simulink model "sf_cruise_control_test"  (R2017b)
settings: Solver=ode45  StartTime=0.0  StopTime=10.0  RelTol=1e-3  EnableMultiTasking=on
PreLoadFcn:
  | Kp = 30; Kd = 30; Ki = 10;
undefined symbols (not defined in the file): DiscIntNeverNeededParam, sigbuilder_block
settings Model: FPTRunName=Active  ExtModeAutoUpdateStatusClock=off  Creator=The MathWorks, Inc.  LastModifiedBy=The MathWorks, Inc.
settings DataIOCC: LimitDataPoints=on  SaveFormat=Array
settings OptimizationCC: BooleanDataType=off  ExpressionDepthLimit=2147483647  InitFltsAndDblsToZero=on  LifeSpan=inf
settings DebuggingCC: SaveWithParameterizedLinksMsg=none  UnderspecifiedInitializationDetection=Classic  MergeDetectMultiDrivingBlocksExec=none  SignalResolutionControl=TryResolveAllWithWarning  MultiTaskDSMMsg=warning  MultiTaskCondExecSysMsg=none  FcnCallInpInsideContextMsg=warning  StateNameClashWarn=warning  StrictBusMsg=None  SFUnexpectedBacktrackingDiag=warning  SFNoUnconditionalDefaultTransitionDiag=warning  SFExecutionAtInitializationDiag=none
settings HardwareCC: ProdBitPerPointer=32  ProdBitPerSizeT=32  ProdBitPerPtrDiffT=32  ProdLargestAtomicFloat=None  ProdIntDivRoundTo=Undefined  ProdEndianess=Unspecified  ProdWordSize=32  ProdHWDeviceType=32-bit Generic  TargetUnknown=on
settings ModelReferenceCC: PropagateSignalLabelsOutOfModel=off
settings SFSimCC: SimParseCustomCode=off
settings CodeAppCC: StateflowObjectComments=on
settings GRTTargetCC: TargetFcnLib=ansi_tfl_tmw.mat  TargetLangStandard=C89/C90 (ANSI)  GeneratePreprocessorConditionals=Disable all  CombineOutputUpdateFcns=off  GRTInterface=on
settings ConfigComp: CovMetricSettings=dcmtr  CovHtmlReporting=on  CovSaveCumulativeToWorkspaceVar=on  CovSaveSingleToWorkspaceVar=on  CovExternalEMLEnable=off  CovSFcnEnable=off

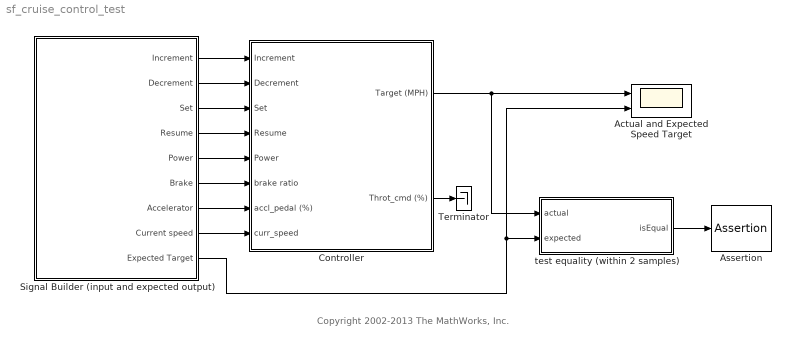
== system sf_cruise_control_test ==
  note: Copyright 2002-2013 The MathWorks, Inc.
  Actual and Expected Speed Target : Scope  NumInputPorts=2
  Assertion : Assertion
  Controller : Subsystem
  Signal Builder (input and expected output) : Subsystem  Tag=STV Subsys  LoadFcn=sigbuilder_block('load');  StartFcn=sigbuilder_block('start');  StopFcn=sigbuilder_block('stop');  ClipboardFcn=sigbuilder_block('clipboard');  mask(Sigbuilder block){tuvar=[0:10]}
      mask init:
      | tuvar = sigbuilder_block('maskInit');
      settings: CopyFcn=sigbuilder_block('copy');  DeleteFcn=sigbuilder_block('delete');  ModelCloseFcn=sigbuilder_block('modelClose');  PreSaveFcn=sigbuilder_block('preSave');  PauseFcn=sigbuilder_block('pause')  ContinueFcn=sigbuilder_block('continue')  NameChangeFcn=sigbuilder_block('namechange');  OpenFcn=sigbuilder_block('open',[41.25 267.75 391.5 268.5 ]);  CloseFcn=sigbuilder_block('close');
      mask Display: plot(0, 0, 100, 100,[2, 2, 32, 32, 2], [68, 8, 8, 68, 68],[32, 2], [38, 38], [32, 19, 2],[53, 60, 44], [32, 17, 17, 2],[16, 16, 31, 31]);txt = getActiveGroup(gcbh);text(2, 100, txt,'verticalAlignment', 'top');
  Terminator : Terminator
  test equality (within 2 samples) : Subsystem
  wires:
  Signal Builder (input and expected output)/1(Increment) -> Controller/1(Increment)
  Signal Builder (input and expected output)/2(Decrement) -> Controller/2(Decrement)
  Signal Builder (input and expected output)/3(Set) -> Controller/3(Set)
  Signal Builder (input and expected output)/4(Resume) -> Controller/4(Resume)
  Signal Builder (input and expected output)/5(Power) -> Controller/5(Power)
  Signal Builder (input and expected output)/6(Brake) -> Controller/6(brake ratio)
  Signal Builder (input and expected output)/7(Accelerator) -> Controller/7(accl_pedal (%))
  Signal Builder (input and expected output)/8(Current speed) -> Controller/8(curr_speed)
  Controller/1(Target (MPH)) -> Actual and Expected Speed Target/1, test equality (within 2 samples)/1(actual)
  Signal Builder (input and expected output)/9(Expected Target) -> test equality (within 2 samples)/2(expected), Actual and Expected Speed Target/2
  test equality (within 2 samples)/1(isEqual) -> Assertion/1
  Controller/2(Throt_cmd (%)) -> Terminator/1

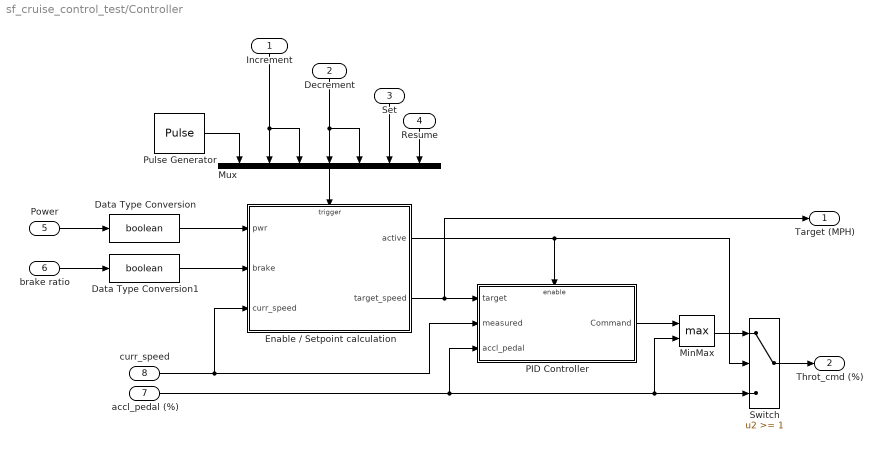
== system sf_cruise_control_test/Controller ==
  Increment : Inport
  Decrement : Inport  Port=2
  Set : Inport  Port=3
  Resume : Inport  Port=4
  Power : Inport  Port=5
  brake ratio : Inport  Port=6
  accl_pedal (%) : Inport  Port=7
  curr_speed : Inport  Port=8
  Data Type Conversion : DataTypeConversion  OutDataTypeStr=boolean
  Data Type Conversion1 : DataTypeConversion  OutDataTypeStr=boolean
  Enable / Setpoint calculation : Stateflow chart  TreatAsAtomicUnit=on
  MinMax : MinMax  Function=max  Inputs=2  ZeroCross=off  SaturateOnIntegerOverflow=on  InputSameDT=on
  Mux : Mux  Inputs=7
  PID Controller : Subsystem  TreatAsAtomicUnit=on
  Pulse Generator : DiscretePulseGenerator  SampleTime=.05
  Switch : Switch  Threshold=1  ZeroCross=off  InputSameDT=on
  Target (MPH) : Outport
  Throt_cmd (%) : Outport  Port=2
  wires:
  Mux/1 -> Enable / Setpoint calculation/Trigger
  Enable / Setpoint calculation/2(target_speed) -> PID Controller/1(target), Target (MPH)/1
  curr_speed/1 -> PID Controller/2(measured), Enable / Setpoint calculation/3(curr_speed)
  accl_pedal (%)/1 -> PID Controller/3(accl_pedal), Switch/3, MinMax/2
  Increment/1 -> Mux/3, Mux/2
  Decrement/1 -> Mux/5, Mux/4
  Set/1 -> Mux/6
  Resume/1 -> Mux/7
  Power/1 -> Data Type Conversion/1
  brake ratio/1 -> Data Type Conversion1/1
  Switch/1 -> Throt_cmd (%)/1
  Enable / Setpoint calculation/1(" active") -> Switch/2, PID Controller/Enable
  MinMax/1 -> Switch/1
  PID Controller/1(Command) -> MinMax/1
  Pulse Generator/1 -> Mux/1
  Data Type Conversion/1 -> Enable / Setpoint calculation/1(pwr)
  Data Type Conversion1/1 -> Enable / Setpoint calculation/2(brake)

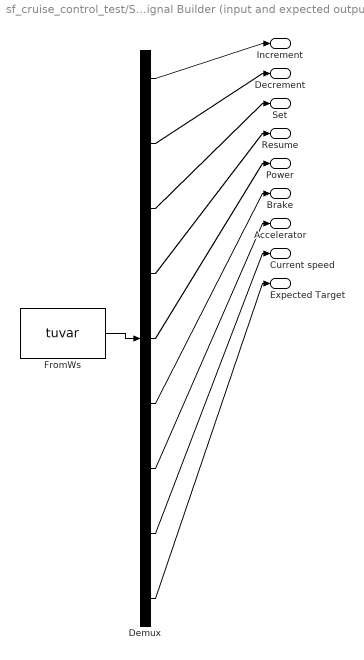
== system sf_cruise_control_test/Signal Builder (input and expected output) ==
  Demux : Demux  Tag=STV Demux  Outputs=9
  FromWs : FromWorkspace  Tag=STV FromWs  VariableName=tuvar  SampleTime=0  OutputAfterFinalValue=Holding final value
      SigBuilderData=|
      | common.afterFinalStr = 'Hold final value'
      | common.sampleTime = 0
      | dataSet(1).timeRange = [0 10]
      | dataSet(1).name = 'Reqs. 1,2,8 (power and set)'
      | dataSet(2).timeRange = [0 10]
      | dataSet(2).name = 'Req. 3 (resume)'
      | dataSet(3).timeRange = [0 10]
      | dataSet(3).name = 'Req. 4 (press inc)'
      | dataSet(4).timeRange = [0 10]
      | dataSet(4).name = 'Req. 5 (hold inc)'
      | dataSet(5).timeRange = [0 10]
      | dataSet(5).name = 'Req. 6 (press dec)'
      | dataSet(6).timeRange = [0 10]
      | dataSet(6).name = 'Req. 7 (hold dec)'
      | dataSet(7).timeRange = [0 10]
      | dataSet(7).name = 'Reqs.9,10 (brake, resume)'
      | sbobj.Groups(1).Name = 'Reqs. 1,2,8 (power and set)'
      | sbobj.Groups(1).Signals(1).Name = 'Increment'
      | sbobj.Groups(1).Signals(1).XData = [0 4 6 10]
      | sbobj.Groups(1).Signals(1).YData = [0 0 0 0]
      | sbobj.Groups(1).Signals(2).Name = 'Decrement'
      | sbobj.Groups(1).Signals(2).XData = [0 10]
      | sbobj.Groups(1).Signals(2).YData = [0 0]
      | sbobj.Groups(1).Signals(3).Name = 'Set'
      | sbobj.Groups(1).Signals(3).XData = [0 3 3 10]
      | sbobj.Groups(1).Signals(3).YData = [0 0 1 1]
      | sbobj.Groups(1).Signals(4).Name = 'Resume'
      | sbobj.Groups(1).Signals(4).XData = [0 10]
      | sbobj.Groups(1).Signals(4).YData = [0 0]
      | sbobj.Groups(1).Signals(5).Name = 'Power'
      | sbobj.Groups(1).Signals(5).XData = [0 1 1 10]
      | sbobj.Groups(1).Signals(5).YData = [0.1 0.1 1 1]
      | sbobj.Groups(1).Signals(6).Name = 'Brake'
      | sbobj.Groups(1).Signals(6).XData = [0 10]
      | sbobj.Groups(1).Signals(6).YData = [0 0]
      | sbobj.Groups(1).Signals(7).Name = 'Accelerator'
      | sbobj.Groups(1).Signals(7).XData = [0 10]
      | sbobj.Groups(1).Signals(7).YData = [0 0]
      | sbobj.Groups(1).Signals(8).Name = 'Current speed'
      | sbobj.Groups(1).Signals(8).XData = [0 10]
      | sbobj.Groups(1).Signals(8).YData = [30 30]
      | sbobj.Groups(1).Signals(9).Name = 'Expected Target'
      | sbobj.Groups(1).Signals(9).XData = [0 3 3 10]
      | sbobj.Groups(1).Signals(9).YData = [0 0 30 30]
      | sbobj.Groups(2).Name = 'Req. 3 (resume)'
      | sbobj.Groups(2).Signals(1).Name = 'Increment'
      | sbobj.Groups(2).Signals(1).XData = [0 4 4 5.2 5.2 6 6 7 7 7.5 7.5 8 8 8.5 8.5 10]
      | sbobj.Groups(2).Signals(1).YData = [0 0 0 0 1 1 0 0 1 1 0 0 1 1 0 0]
      | sbobj.Groups(2).Signals(2).Name = 'Decrement'
      | sbobj.Groups(2).Signals(2).XData = [0 10]
      | sbobj.Groups(2).Signals(2).YData = [0 0]
      | sbobj.Groups(2).Signals(3).Name = 'Set'
      | sbobj.Groups(2).Signals(3).XData = [0 3 3 10]
      | sbobj.Groups(2).Signals(3).YData = [0 0 1 1]
      | sbobj.Groups(2).Signals(4).Name = 'Resume'
      | sbobj.Groups(2).Signals(4).XData = [0 9 9 10]
      | sbobj.Groups(2).Signals(4).YData = [0 0 1 1]
      | sbobj.Groups(2).Signals(5).Name = 'Power'
      | sbobj.Groups(2).Signals(5).XData = [0 1 1 10]
      | sbobj.Groups(2).Signals(5).YData = [0.1 0.1 1 1]
      | sbobj.Groups(2).Signals(6).Name = 'Brake'
      | sbobj.Groups(2).Signals(6).XData = [0 10]
      | sbobj.Groups(2).Signals(6).YData = [0 0]
      | sbobj.Groups(2).Signals(7).Name = 'Accelerator'
      | sbobj.Groups(2).Signals(7).XData = [0 10]
      | sbobj.Groups(2).Signals(7).YData = [0 0]
      | sbobj.Groups(2).Signals(8).Name = 'Current speed'
      | sbobj.Groups(2).Signals(8).XData = [0 10]
      | sbobj.Groups(2).Signals(8).YData = [30 30]
      | sbobj.Groups(2).Signals(9).Name = 'Expected Target'
      | sbobj.Groups(2).Signals(9).XData = [0 3 3 5.2 5.2 7 7 8 8 9 9 10]
      | sbobj.Groups(2).Signals(9).YData = [0 0 30 30 31 31 32 32 33 33 30 30]
      | sbobj.Groups(3).Name = 'Req. 4 (press inc)'
      | sbobj.Groups(3).Signals(1).Name = 'Increment'
      | sbobj.Groups(3).Signals(1).XData = [0 4 5.2 5.2 6 6 7 7 7.5 7.5 8 8 8.5 8.5 10]
      | sbobj.Groups(3).Signals(1).YData = [0 0 0 1 1 0 0 1 1 0 0 1 1 0 0]
      | sbobj.Groups(3).Signals(2).Name = 'Decrement'
      | sbobj.Groups(3).Signals(2).XData = [0 10]
      | sbobj.Groups(3).Signals(2).YData = [0 0]
      | sbobj.Groups(3).Signals(3).Name = 'Set'
      | sbobj.Groups(3).Signals(3).XData = [0 3 3 10]
      | sbobj.Groups(3).Signals(3).YData = [0 0 1 1]
      | sbobj.Groups(3).Signals(4).Name = 'Resume'
      | sbobj.Groups(3).Signals(4).XData = [0 10]
      | sbobj.Groups(3).Signals(4).YData = [0 0]
      | sbobj.Groups(3).Signals(5).Name = 'Power'
      | sbobj.Groups(3).Signals(5).XData = [0 1 1 10]
      | sbobj.Groups(3).Signals(5).YData = [0.1 0.1 1 1]
      | sbobj.Groups(3).Signals(6).Name = 'Brake'
      | sbobj.Groups(3).Signals(6).XData = [0 10]
      | sbobj.Groups(3).Signals(6).YData = [0 0]
      | sbobj.Groups(3).Signals(7).Name = 'Accelerator'
      | sbobj.Groups(3).Signals(7).XData = [0 10]
      | sbobj.Groups(3).Signals(7).YData = [0 0]
      | sbobj.Groups(3).Signals(8).Name = 'Current speed'
      | sbobj.Groups(3).Signals(8).XData = [0 10]
      | sbobj.Groups(3).Signals(8).YData = [30 30]
      | sbobj.Groups(3).Signals(9).Name = 'Expected Target'
      | sbobj.Groups(3).Signals(9).XData = [0 3 3 5.2 5.2 7 7 8 8 9 10]
      | sbobj.Groups(3).Signals(9).YData = [0 0 30 30 31 31 32 32 33 33 33]
      | sbobj.Groups(4).Name = 'Req. 5 (hold inc)'
      | sbobj.Groups(4).Signals(1).Name = 'Increment'
      | sbobj.Groups(4).Signals(1).XData = [0 3 3 9.5 9.5 10]
      | sbobj.Groups(4).Signals(1).YData = [0 0 1 1 0 0]
      | sbobj.Groups(4).Signals(2).Name = 'Decrement'
      | sbobj.Groups(4).Signals(2).XData = [0 10]
      | sbobj.Groups(4).Signals(2).YData = [0 0]
      | sbobj.Groups(4).Signals(3).Name = 'Set'
      | sbobj.Groups(4).Signals(3).XData = [0 2 2 10]
      | sbobj.Groups(4).Signals(3).YData = [0 0 1 1]
      | sbobj.Groups(4).Signals(4).Name = 'Resume'
      | sbobj.Groups(4).Signals(4).XData = [0 10]
      | sbobj.Groups(4).Signals(4).YData = [0 0]
      | sbobj.Groups(4).Signals(5).Name = 'Power'
      | sbobj.Groups(4).Signals(5).XData = [0 1 1 10]
      | sbobj.Groups(4).Signals(5).YData = [0.1 0.1 1 1]
      | sbobj.Groups(4).Signals(6).Name = 'Brake'
      | sbobj.Groups(4).Signals(6).XData = [0 10]
      | sbobj.Groups(4).Signals(6).YData = [0 0]
      | sbobj.Groups(4).Signals(7).Name = 'Accelerator'
      | sbobj.Groups(4).Signals(7).XData = [0 10]
      | sbobj.Groups(4).Signals(7).YData = [0 0]
      | sbobj.Groups(4).Signals(8).Name = 'Current speed'
      | sbobj.Groups(4).Signals(8).XData = [0 10]
      | sbobj.Groups(4).Signals(8).YData = [30 30]
      | sbobj.Groups(4).Signals(9).Name = 'Expected Target'
      | sbobj.Groups(4).Signals(9).XData = [0 2 2 3 3 4 4 5 5 6 6 7 7 8 8 9 9 10]
      | sbobj.Groups(4).Signals(9).YData = [0 0 30 30 31 31 32 32 33 33 34 34 35 35 36 36 37 37]
      | sbobj.Groups(5).Name = 'Req. 6 (press dec)'
      | sbobj.Groups(5).Signals(1).Name = 'Increment'
      | sbobj.Groups(5).Signals(1).XData = [0 10]
      | sbobj.Groups(5).Signals(1).YData = [0 0]
      | sbobj.Groups(5).Signals(2).Name = 'Decrement'
      | sbobj.Groups(5).Signals(2).XData = [0 4 5.2 5.2 6 6 7 7 7.5 7.5 8 8 8.5 8.5 10]
      | sbobj.Groups(5).Signals(2).YData = [0 0 0 1 1 0 0 1 1 0 0 1 1 0 0]
      | sbobj.Groups(5).Signals(3).Name = 'Set'
      | sbobj.Groups(5).Signals(3).XData = [0 3 3 10]
      | sbobj.Groups(5).Signals(3).YData = [0 0 1 1]
      | sbobj.Groups(5).Signals(4).Name = 'Resume'
      | sbobj.Groups(5).Signals(4).XData = [0 10]
      | sbobj.Groups(5).Signals(4).YData = [0 0]
      | sbobj.Groups(5).Signals(5).Name = 'Power'
      | sbobj.Groups(5).Signals(5).XData = [0 1 1 10]
      | sbobj.Groups(5).Signals(5).YData = [0.1 0.1 1 1]
      | sbobj.Groups(5).Signals(6).Name = 'Brake'
      | sbobj.Groups(5).Signals(6).XData = [0 10]
      | sbobj.Groups(5).Signals(6).YData = [0 0]
      | sbobj.Groups(5).Signals(7).Name = 'Accelerator'
      | sbobj.Groups(5).Signals(7).XData = [0 10]
      | sbobj.Groups(5).Signals(7).YData = [0 0]
      | sbobj.Groups(5).Signals(8).Name = 'Current speed'
      | sbobj.Groups(5).Signals(8).XData = [0 10]
      | sbobj.Groups(5).Signals(8).YData = [30 30]
      | sbobj.Groups(5).Signals(9).Name = 'Expected Target'
      | sbobj.Groups(5).Signals(9).XData = [0 3 3 5.2 5.2 7 7 8 8 9 10]
      | sbobj.Groups(5).Signals(9).YData = [0 0 30 30 29 29 28 28 27 27 27]
      | sbobj.Groups(6).Name = 'Req. 7 (hold dec)'
      | sbobj.Groups(6).Signals(1).Name = 'Increment'
      | sbobj.Groups(6).Signals(1).XData = [0 10]
      | sbobj.Groups(6).Signals(1).YData = [0 0]
      | sbobj.Groups(6).Signals(2).Name = 'Decrement'
      | sbobj.Groups(6).Signals(2).XData = [0 3 3 9.5 9.5 10]
      | sbobj.Groups(6).Signals(2).YData = [0 0 1 1 0 0]
      | sbobj.Groups(6).Signals(3).Name = 'Set'
      | sbobj.Groups(6).Signals(3).XData = [0 2 2 10]
      | sbobj.Groups(6).Signals(3).YData = [0 0 1 1]
      | sbobj.Groups(6).Signals(4).Name = 'Resume'
      | sbobj.Groups(6).Signals(4).XData = [0 10]
      | sbobj.Groups(6).Signals(4).YData = [0 0]
      | sbobj.Groups(6).Signals(5).Name = 'Power'
      | sbobj.Groups(6).Signals(5).XData = [0 1 1 10]
      | sbobj.Groups(6).Signals(5).YData = [0.1 0.1 1 1]
      | sbobj.Groups(6).Signals(6).Name = 'Brake'
      | sbobj.Groups(6).Signals(6).XData = [0 10]
      | sbobj.Groups(6).Signals(6).YData = [0 0]
      | sbobj.Groups(6).Signals(7).Name = 'Accelerator'
      | sbobj.Groups(6).Signals(7).XData = [0 10]
      | sbobj.Groups(6).Signals(7).YData = [0 0]
      | sbobj.Groups(6).Signals(8).Name = 'Current speed'
      | sbobj.Groups(6).Signals(8).XData = [0 10]
      | sbobj.Groups(6).Signals(8).YData = [30 30]
      | sbobj.Groups(6).Signals(9).Name = 'Expected Target'
      | sbobj.Groups(6).Signals(9).XData = [0 2 2 3 3 4 4 5 5 6 6 7 7 8 8 9 9 10]
      | sbobj.Groups(6).Signals(9).YData = [0 0 30 30 29 29 28 28 27 27 26 26 25 25 24 24 23 23]
      | sbobj.Groups(7).Name = 'Reqs.9,10 (brake, resume)'
      | sbobj.Groups(7).Signals(1).Name = 'Increment'
      | sbobj.Groups(7).Signals(1).XData = [0 4 6 10]
      | sbobj.Groups(7).Signals(1).YData = [0 0 0 0]
      | sbobj.Groups(7).Signals(2).Name = 'Decrement'
      | sbobj.Groups(7).Signals(2).XData = [0 10]
      | sbobj.Groups(7).Signals(2).YData = [0 0]
      | sbobj.Groups(7).Signals(3).Name = 'Set'
      | sbobj.Groups(7).Signals(3).XData = [0 0.98 0.98 4.02 4.02 10]
      | sbobj.Groups(7).Signals(3).YData = [0 0 1 1 0 0]
      | sbobj.Groups(7).Signals(4).Name = 'Resume'
      | sbobj.Groups(7).Signals(4).XData = [0 7 7 10]
      | sbobj.Groups(7).Signals(4).YData = [0 0 1 1]
      | sbobj.Groups(7).Signals(5).Name = 'Power'
      | sbobj.Groups(7).Signals(5).XData = [0 0.52 0.52 10]
      | sbobj.Groups(7).Signals(5).YData = [0.1 0.1 1 1]
      | sbobj.Groups(7).Signals(6).Name = 'Brake'
      | sbobj.Groups(7).Signals(6).XData = [0 3 3 3.5 3.5 5 5 5.5 5.5 10]
      | sbobj.Groups(7).Signals(6).YData = [0 0 0.7 0.7 0 0 0.7 0.7 0 0]
      | sbobj.Groups(7).Signals(7).Name = 'Accelerator'
      | sbobj.Groups(7).Signals(7).XData = [0 10]
      | sbobj.Groups(7).Signals(7).YData = [0 0]
      | sbobj.Groups(7).Signals(8).Name = 'Current speed'
      | sbobj.Groups(7).Signals(8).XData = [0 10]
      | sbobj.Groups(7).Signals(8).YData = [30 30]
      | sbobj.Groups(7).Signals(9).Name = 'Expected Target'
      | sbobj.Groups(7).Signals(9).XData = [0 1 1 3 3 4 4 5 5 7 7 10]
      | sbobj.Groups(7).Signals(9).YData = [0 0 30 30 0 0 30 30 0 0 30 30]
  Increment : Outport  Tag=STV Outport
  Decrement : Outport  Tag=STV Outport  Port=2
  Set : Outport  Tag=STV Outport  Port=3
  Resume : Outport  Tag=STV Outport  Port=4
  Power : Outport  Tag=STV Outport  Port=5
  Brake : Outport  Tag=STV Outport  Port=6
  Accelerator : Outport  Tag=STV Outport  Port=7
  Current speed : Outport  Tag=STV Outport  Port=8
  Expected Target : Outport  Tag=STV Outport  Port=9
  wires:
  Demux/9 -> Expected Target/1
  Demux/8 -> Current speed/1
  Demux/7 -> Accelerator/1
  Demux/6 -> Brake/1
  Demux/5 -> Power/1
  Demux/4 -> Resume/1
  Demux/3 -> Set/1
  Demux/2 -> Decrement/1
  Demux/1 -> Increment/1
  FromWs/1 -> Demux/1

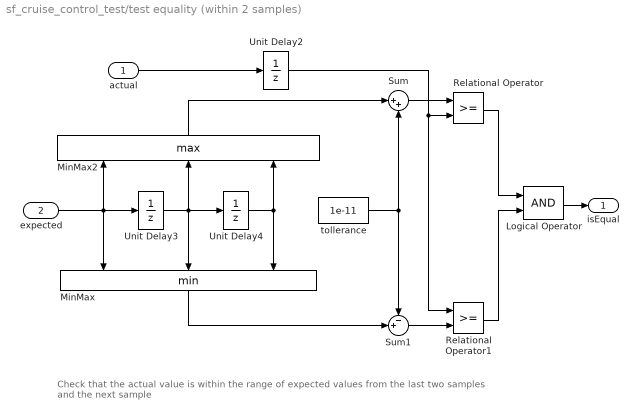
== system sf_cruise_control_test/test equality (within 2 samples) ==
  note: Check that the actual value is within the range of expected
      | values from the last two samples and the next sample
  actual : Inport
  expected : Inport  Port=2
  Logical Operator : Logic
  MinMax : MinMax  Inputs=3  ZeroCross=off  SaturateOnIntegerOverflow=on  InputSameDT=on
  MinMax2 : MinMax  Function=max  Inputs=3  ZeroCross=off  SaturateOnIntegerOverflow=on  InputSameDT=on
  Relational Operator : RelationalOperator  ZeroCross=off  RndMeth=Nearest  InputSameDT=on
  Relational Operator1 : RelationalOperator  ZeroCross=off  RndMeth=Nearest  InputSameDT=on
  Sum : Sum  Inputs=|++  SaturateOnIntegerOverflow=on  InputSameDT=on  OutDataTypeStr=Inherit: Same as first input
  Sum1 : Sum  Inputs=-+|  SaturateOnIntegerOverflow=on  InputSameDT=on  OutDataTypeStr=Inherit: Same as first input
  Unit Delay2 : UnitDelay  SampleTime=0.1
  Unit Delay3 : UnitDelay  SampleTime=0.1
  Unit Delay4 : UnitDelay  SampleTime=0.1
  tollerance : Constant  Value=1e-11
  isEqual : Outport
  wires:
  Logical Operator/1 -> isEqual/1
  actual/1 -> Unit Delay2/1
  Relational Operator1/1 -> Logical Operator/2
  Relational Operator/1 -> Logical Operator/1
  expected/1 -> Unit Delay3/1, MinMax/1, MinMax2/1
  Unit Delay3/1 -> Unit Delay4/1, MinMax/2, MinMax2/2
  Unit Delay2/1 -> Relational Operator1/1, Relational Operator/2
  Unit Delay4/1 -> MinMax2/3, MinMax/3
  MinMax2/1 -> Sum/1
  Sum/1 -> Relational Operator/1
  Sum1/1 -> Relational Operator1/2
  MinMax/1 -> Sum1/2
  tollerance/1 -> Sum1/1, Sum/2

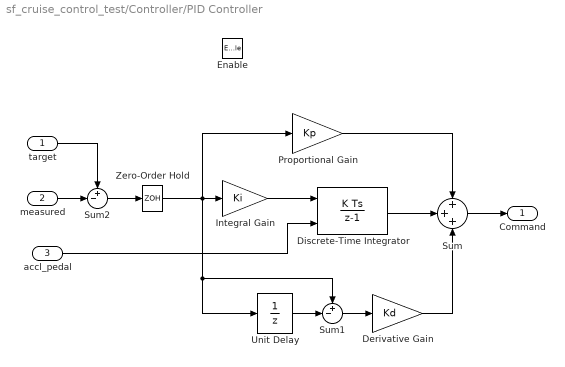
== system sf_cruise_control_test/Controller/PID Controller ==
  target : Inport
  measured : Inport  Port=2
  accl_pedal : Inport  Port=3
  Enable : EnablePort  StatesWhenEnabling=reset  ZeroCross=off
  Derivative Gain : Gain  Gain=Kd  SaturateOnIntegerOverflow=on  OutDataTypeStr=Inherit: Same as input  ParamDataTypeStr=Inherit: Same as input
  Discrete-Time Integrator : DiscreteIntegrator  InitialConditionSource=external  SampleTime=0.1  UpperSaturationLimit=20  LowerSaturationLimit=-20  ICPrevOutput=DiscIntNeverNeededParam  ICPrevScaledInput=DiscIntNeverNeededParam
  Integral Gain : Gain  Gain=Ki  SaturateOnIntegerOverflow=on  OutDataTypeStr=Inherit: Same as input  ParamDataTypeStr=Inherit: Same as input
  Proportional Gain : Gain  Gain=Kp  SaturateOnIntegerOverflow=on  OutDataTypeStr=Inherit: Same as input  ParamDataTypeStr=Inherit: Same as input
  Sum : Sum  Inputs=+++  SaturateOnIntegerOverflow=on  InputSameDT=on  OutDataTypeStr=Inherit: Same as first input
  Sum1 : Sum  Inputs=+-|  SaturateOnIntegerOverflow=on  InputSameDT=on  OutDataTypeStr=Inherit: Same as first input
  Sum2 : Sum  Inputs=+-|  SaturateOnIntegerOverflow=on  InputSameDT=on  OutDataTypeStr=Inherit: Same as first input
  Unit Delay : UnitDelay  SampleTime=0.1
  Zero-Order Hold : ZeroOrderHold  SampleTime=0.1
  Command : Outport
  wires:
  Unit Delay/1 -> Sum1/2
  Sum1/1 -> Derivative Gain/1
  Discrete-Time Integrator/1 -> Sum/2
  Derivative Gain/1 -> Sum/3
  Proportional Gain/1 -> Sum/1
  Sum2/1 -> Zero-Order Hold/1
  Sum/1 -> Command/1
  target/1 -> Sum2/1
  measured/1 -> Sum2/2
  Integral Gain/1 -> Discrete-Time Integrator/1
  accl_pedal/1 -> Discrete-Time Integrator/2
  Zero-Order Hold/1 -> Proportional Gain/1, Unit Delay/1, Sum1/1, Integral Gain/1

== stateflow chart sf_cruise_control_test/Controller/Enable / Setpoint calculation ==
  state Set_Point_Calculation [parallel]
    settings: executionOrder=1
    state Decrement
      en: target_speed--;
      Decrement -> Decrement [order 1] : every(10,Update)
          | {target_speed--;}
    state Increment
      en: target_speed++;
      Increment -> Increment [order 1] : every(10,Update)
          | {target_speed++;}
    state Hold
      Hold -> (junction 30) [order 2] : Resume [pwr]
      Hold -> (junction 29) [order 1] : Set [pwr]
          | {
          | target_speed = curr_speed;
          | set_speed = curr_speed;
          | }
      (junction 30) -> (junction 31) [order 2]
      (junction 30) -> (junction 31) [order 1] : [set_speed > 0]
          |
          | {target_speed = ...
          | set_speed;}
    (default) -> Hold
    Decrement -> Hold [order 1] : DEC_BU
    Increment -> Hold [order 1] : INC_BU
    Hold -> Decrement [order 1] : DEC_BD
        | [in(Enable.on.active)]
    Hold -> Increment [order 2] : INC_BD
        | [in(Enable.on.active)]
  state Enable [parallel]
    settings: executionOrder=2
    state on
      state overide
        target_speed = 0;
      state no_target
      state active
      (default) -> no_target
      overide -> active : Set | Resume
      active -> overide : [brake]
      no_target -> active : Set
    state Off
    (default) -> Off
    on -> Off : [!pwr]
    Off -> on : [pwr]
  data: pwr input boolean; brake input boolean; active output boolean; target_speed output double; set_speed local double; curr_speed input double
  events: Update input RISING_EDGE_EVENT; INC_BD input RISING_EDGE_EVENT; INC_BU input FALLING_EDGE_EVENT; DEC_BD input RISING_EDGE_EVENT; DEC_BU input FALLING_EDGE_EVENT; Set input EITHER_EDGE_EVENT; Resume input EITHER_EDGE_EVENT
